simulink model "UnitTest_Breaker_EGC"  (Simulink 8.1)
settings: Solver=ode4  StartTime=0.0  StopTime=8  FixedStep=Ts  MaxStep=1e-3  RelTol=1e-3
model workspace (MAT data in the model file):
  op_snapshot1 : opcond.OperatingPoint (value not decoded)
PostLoadFcn:
  | Ts=100e-6; UnitTest_Breaker_init;
InitFcn:
  | Ts=100e-6; UnitTest_Breaker_init;
undefined symbols (not defined in the file or in its folder): cb_mech_delay
libraries: powerlib x3, Load_lib x2, simulink x2, artemis x1, breaker_lib x1, rtlab x1, cables_lib x1, transformer_lib x1
settings Model: ARTEMISmethode_block_infos=$$__separator__$$UnitTest_Breaker_EGC/ARTEMIS Guide$$__separator__$$  Creator=RE25624  LastModifiedBy=ed12083  BufferReuse=off
settings SolverCC: ZeroCrossAlgorithm=Adaptive
settings DataIOCC: ExternalInput=getinputstruct(op_snapshot1)  InitialState=getstatestruct(op_snapshot1)  LimitDataPoints=off  MaxDataPoints=90060  SignalLoggingSaveFormat=Dataset  SaveOutput=off  SignalLogging=off  DSMLogging=off  SaveTime=off  OutputSaveName=result
settings OptimizationCC: BlockReduction=off  OptimizeBlockIOStorage=off  BufferReuse=off  ExpressionFolding=off  LocalBlockOutputs=off
settings DebuggingCC: MaxConsecutiveZCsMsg=warning  IgnoredZcDiagnostic=none  SolverPrmCheckMsg=none  MultiTaskRateTransMsg=warning  FcnCallInpInsideContextMsg=EnableAllAsWarning  FrameProcessingCompatibilityMsg=error  ModelReferenceExtraNoncontSigs=warning  StrictBusMsg=None
settings ModelReferenceCC: UpdateModelReferenceTargets=IfOutOfDate
settings SFSimCC: SFSimEcho=off
settings GRTTargetCC: CodeReplacementLibrary=C89/C90 (ANSI)

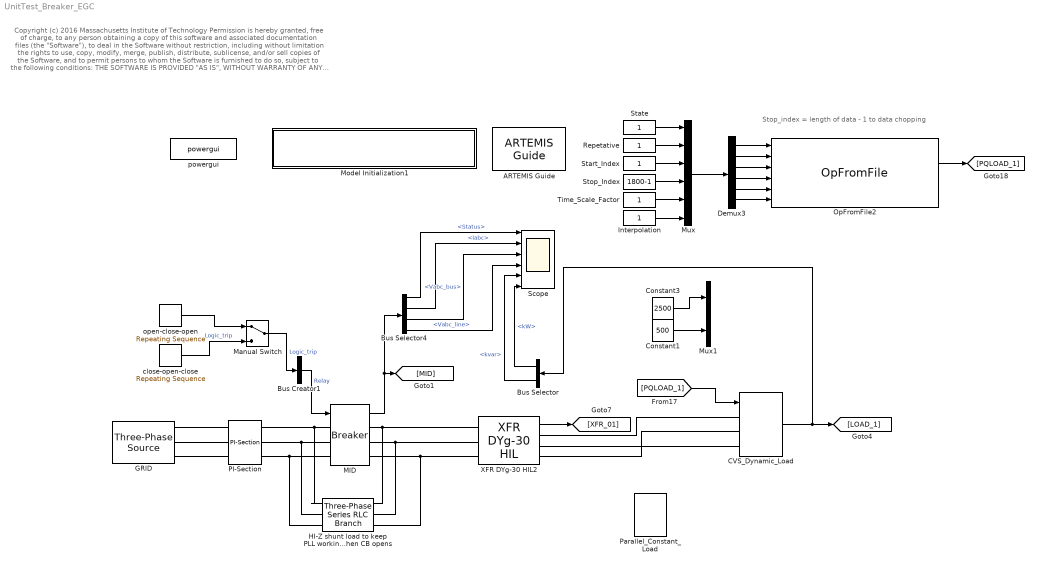
== system UnitTest_Breaker_EGC ==
  note: Copyright (c) 2016 Massachusetts Institute of Technology
      | Permission is hereby granted, free of charge, to any person obtaining a copy of this software and associated documentation files (the "Software"), to deal
      | in the Software without restriction, including without limitation the rights to use, copy, modify, merge, publish, distribute, sublicense, and/or sell copies of the
      | Software, and to permit persons to whom the Software is furnished to do so, subject to the following conditions:
      |
      | THE SOFTWARE IS PROVIDED "AS IS", WITHOUT WARRANTY OF ANY KIND, EXPRESS OR IMPLIED, INCLUDING BUT NOT LIMITED TO THE
      | WARRANTIES OF MERCHANTABILITY, FITNESS FOR A PARTICULAR PURPOSE AND NONINFRINGEMENT. IN NO EVENT SHALL THE AUTHORS
      | OR COPYRIGHT HOLDERS BE LIABLE FOR ANY CLAIM, DAMAGES OR OTHER LIABILITY, WHETHER IN AN ACTION OF CONTRACT, TORT OR
      | OTHERWISE, ARISING FROM, OUT OF OR IN CONNECTION WITH THE SOFTWARE OR THE USE OR OTHER DEALINGS IN THE SOFTWARE.
  note: Stop_index = length of data - 1 to data chopping
  ARTEMIS Guide : artemis/ARTEMIS/ARTEMIS Guide  Tag=FTSSmethode_opal_4hx0r99  Description=5.0_z1  lock=on  Ts=Ts  opt=art5  dyna=off  nb_perm=4  RT_fullcomp=off  ssn=on  ssn_itvc=off  ssn_ivic=off  ssn_ext=off  ssn_solver=Art5 with Backward Euler nodal interface  ssn_impulse=off  ssn_quasimpulse=off  ssn_impulse_loop=2  paraExtinctionThy=off  Thy_Impulse=on  dtc=Off  dtc_opt=normal  ao=on  simtype=off  ct_mac=off  lin_mov=off  lsp=[0.001 2]  spike_skip=Disabled  dtc_extra=1  dtc_sws=normal  dtc_pied=0.5  SPSRulesBlock=SPSRules  tre=on  ctmm=off  LF=off  dpl_type=ARTEMiS DPL  rlc_type=off  custom_type=off  para=on  ssn_ImpulseLoopBlockedStateUpdate=2  ssn_mov_iter_number=5  ssn_switch_iter_number=5
  Bus Creator1 : BusCreator  Inputs=1
  Bus Selector : BusSelector  OutputSignals=kW,kvar
  Bus Selector4 : BusSelector  OutputSignals=Status,Iabc,Vabc_bus,Vabc_line
  CVS_Dynamic_Load : Load_lib/CVS_Dynamic_Load  V=480  Ts=Ts
  Constant1 : Constant  Value=500
  Constant3 : Constant  Value=2500
  Demux3 : Demux  Outputs=6
  GRID : powerlib/Electrical Sources/Three-Phase Source  Voltage=13800  PhaseAngle=0  Frequency=60  InternalConnection=Yg  SpecifyImpedance=on  Resistance=0.8929  Inductance=16.58e-3  ShortCircuitLevel=375e6  BaseVoltage=13800  XRratio=7.9  BusType=swing  Pref=0  Qref=0  Qmin=-inf  Qmax=inf
  "HI-Z shunt load to keep PLL working when CB opens " : powerlib/Elements/Three-Phase Series RLC Branch  LConnTagsString=A|B|C  RConnTagsString=A|B|C  BranchType=RLC  Resistance=10e6  Inductance=0  Capacitance=inf  Measurements=None
  "Interpolation " : Constant
  MID : breaker_lib/Breaker  Ts=Ts  mech_delays=[cb_mech_delay(1,:)]
  Manual Switch : ManualSwitch
  Model Initialization1 : Subsystem  AncestorBlock=artemis/Tools /Misc/Model Initialization  mask(Model Functions){InitFcnX=Ts=100e-6; UnitTest_Breaker_init;, prel=off, posl=on, inif=on, strf=off}
      mask prompts: InitFcnX "Initialisation"; prel "Preload Function"; posl "PostLoad Function"; inif "InitFcn"; strf "StartFcn"
      mask init:
      | currentBlock = gcb;
      | root = bdroot(currentBlock);
      | 
      | 
      | if ~strcmp(get_param(root,'BlockDiagramType'),'library')
      |     if prel==1
      |         set_param(root, 'PreLoadFcn', InitFcnX);
      |     else
      |         set_param(root, 'PreLoadFcn', '');
      |     end
      |     if inif==1
      |         set_param(root, 'InitFcn', InitFcnX);
      |     else
      |         set_param(root, 'InitFcn', '');
      |     end
      |     if strf==1
      |         set_param(root, 'StartFcn', InitFcnX);
      |     else
      |         set_param(root, 'StartFcn', '');
      |     end
      |     if posl==1
      |         set_param(root, 'PostLoadFcn', InitFcnX);
      |     else
      |         set_param(root, 'PostLoadFcn', '');
      |     end
      | end
      | 
      | pos = get_param(currentBlock, 'Position');
      | width = pos(3) - pos(1); height = pos(4) - pos(2);
      | txt = [ upper(root) '\n' '- InitFcn. . . . . '  get_param(root, 'InitFcn') ];
      settings: CopyFcn=set_param(gcb,'LinkStatus','inactive')
      mask Display: text(5, height*0.5, txt, 'horizontalAlignment', 'left', 'verticalAlignment', 'middle') ;
  Mux : Mux  Inputs=6
  Mux1 : Mux  Inputs=2
  OpFromFile2 : rtlab/DataLogging/OpFromFile  filename_mode=Static (same filename all the time)  reload_mode=Next time model is paused (Real-Time)  init_file_id=0  filename=one_min_data.mat  rtpath='./'  nrtpath='..\CHPandThermal\'  sample_time=0
  PI-Section : cables_lib/PI-Section  cable_spec=[0.074938, 1.1405, 0.00030953, 0.002005, 6.3294e-07, 6.3294e-07]  line_length=10000  parallel_sets=1
  Parallel_Constant_Load : Load_lib/Parallel_Constant_Load  v=480  kVA=500  pf=0.90
  "Repetative " : Constant
  Scope : Scope  NumInputPorts=6
      settings: TimeRange=8  YMin=0~-200~-12500~-12500~-50~-250  YMax=1~200~12500~12500~550~2750  SaveName=ScopeData2
  "Start_Index " : Constant
  "State " : Constant
  "Stop_Index " : Constant  Value=1800-1
  "Time_Scale_Factor " : Constant
  XFR DYg-30 HIL2 : transformer_lib/XFR DYg-30 HIL  Rating=2500  Vp=13800  Vs=480  Z=5.75  XR=6.6
  close-open-close : simulink/Sources/Repeating Sequence  rep_seq_t=[0 2.5 2.5 4.5 4.5 10]  rep_seq_y=[1 1 0 0 1 1]
  open-close-open : simulink/Sources/Repeating Sequence  rep_seq_t=[0 2.5 2.5 4.5 4.5 10]  rep_seq_y="[0 1  1 1 0 0]"
  powergui : powerlib/powergui  Priority=2  SimulationMode=Discrete  SolverType=Tustin  SampleTime=Ts  frequency=60  SPID=off  DisableSnubberDevices=off  DisableRonSwitches=off  DisableVfSwitches=off  SwTol=0  Interpol=off  DisplayEquations=off  frequencyindice=0  Pbase=100e6  ErrMax=1e-4  Iterations=50  UnitsV=kV  UnitsW=MW  FunctionMessages=off  echomessages=off  HookPort=off  EnableUseOfTLC=off  x0status=blocks  RestoreLinks=warning  ResistiveCurrentMeasurement=off  Frange=logspace(0,3,50)  Ylog=off  Xlog=off  ShowGrid=off  save=off  variable=ZData  structure=0  ZoomFFT=on  StartTime=0.0  cycles=2  DisplayStyle=off  fundamental=60  FreqAxis=off  MaxFrequency=1000  frequencyindicesteady=1  RmsSteady=1  display=off  Ts=0  methode=off
  wires:
  MID/1 -> [MID], Bus Selector4/1
  XFR DYg-30 HIL2/1 -> [XFR_01]
  CVS_Dynamic_Load/1 -> Bus Selector/1, [LOAD_1]
  "Stop_Index "/1 -> Mux/4
  "Interpolation "/1 -> Mux/6
  "Start_Index "/1 -> Mux/3
  "Time_Scale_Factor "/1 -> Mux/5
  "Repetative "/1 -> Mux/2
  "State "/1 -> Mux/1
  Demux3/2 -> OpFromFile2/2
  Demux3/5 -> OpFromFile2/5
  OpFromFile2/2 -> [PQLOAD_1]
  Demux3/4 -> OpFromFile2/4
  Demux3/1 -> OpFromFile2/1
  Demux3/6 -> OpFromFile2/6
  Demux3/3 -> OpFromFile2/3
  Mux/1 -> Demux3/1
  Bus Creator1/1 -> MID/1  "Relay"
  Bus Selector4/1 -> Scope/1  "<Status>"
  Bus Selector4/2 -> Scope/2  "<Iabc>"
  Bus Selector4/3 -> Scope/3  "<Vabc_bus>"
  Bus Selector4/4 -> Scope/4  "<Vabc_line>"
  open-close-open/1 -> Manual Switch/1
  close-open-close/1 -> Manual Switch/2  "Logic_trip"
  Manual Switch/1 -> Bus Creator1/1  "Logic_trip"
  Bus Selector/1 -> Scope/6  "<kW>"
  Bus Selector/2 -> Scope/5  "<kvar>"
  Constant3/1 -> Mux1/1
  Constant1/1 -> Mux1/2
  [PQLOAD_1] -> CVS_Dynamic_Load/1
  connections:
  XFR DYg-30 HIL2/LConn3 -- "HI-Z shunt load to keep PLL working when CB opens "/RConn3 -- MID/RConn3
  XFR DYg-30 HIL2/LConn2 -- "HI-Z shunt load to keep PLL working when CB opens "/RConn2 -- MID/RConn2
  XFR DYg-30 HIL2/LConn1 -- "HI-Z shunt load to keep PLL working when CB opens "/RConn1 -- MID/RConn1
  CVS_Dynamic_Load/LConn2 -- XFR DYg-30 HIL2/RConn2
  CVS_Dynamic_Load/LConn3 -- XFR DYg-30 HIL2/RConn3
  CVS_Dynamic_Load/LConn1 -- XFR DYg-30 HIL2/RConn1
  PI-Section/RConn1 -- "HI-Z shunt load to keep PLL working when CB opens "/LConn1 -- MID/LConn1
  PI-Section/RConn3 -- "HI-Z shunt load to keep PLL working when CB opens "/LConn3 -- MID/LConn3
  PI-Section/RConn2 -- "HI-Z shunt load to keep PLL working when CB opens "/LConn2 -- MID/LConn2
  PI-Section/LConn3 -- GRID/RConn3
  PI-Section/LConn2 -- GRID/RConn2
  PI-Section/LConn1 -- GRID/RConn1

== system UnitTest_Breaker_EGC/Model Initialization1 ==
